simulink model "CraneModel"  (R2021b)
settings: Solver=VariableStepAuto  StartTime=0.0  StopTime=20  MaxStep=0.0001  RelTol=1e-3
values from neighbouring files (symbols this model uses):
  B_x = 12    [variables.m]
  cFrictionX = 18    [variables.m]
  InitWireLength = 1    [variables.m]
  InitXPos = 0    [variables.m]
  J_x = 0.13    [variables.m]
  k_ex = 0.609    [variables.m]
  m_l = 3.89    [variables.m]
  m_t = 0.729    [variables.m]
  r_x = 0.075    [variables.m]
  sFrictionX = 20    [variables.m]
settings Model: Creator=laula  LastModifiedBy=bosto

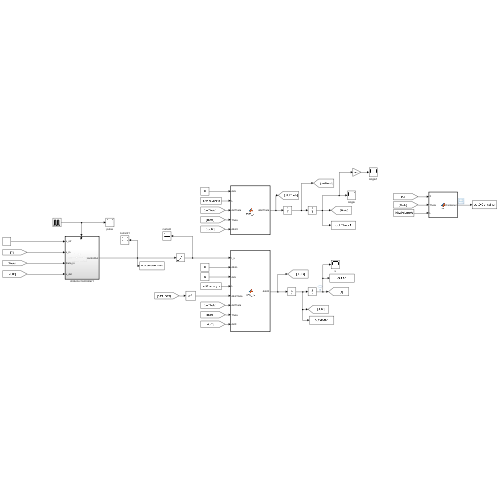
[thumbnail: Simulink's stored preview of the top-level diagram]
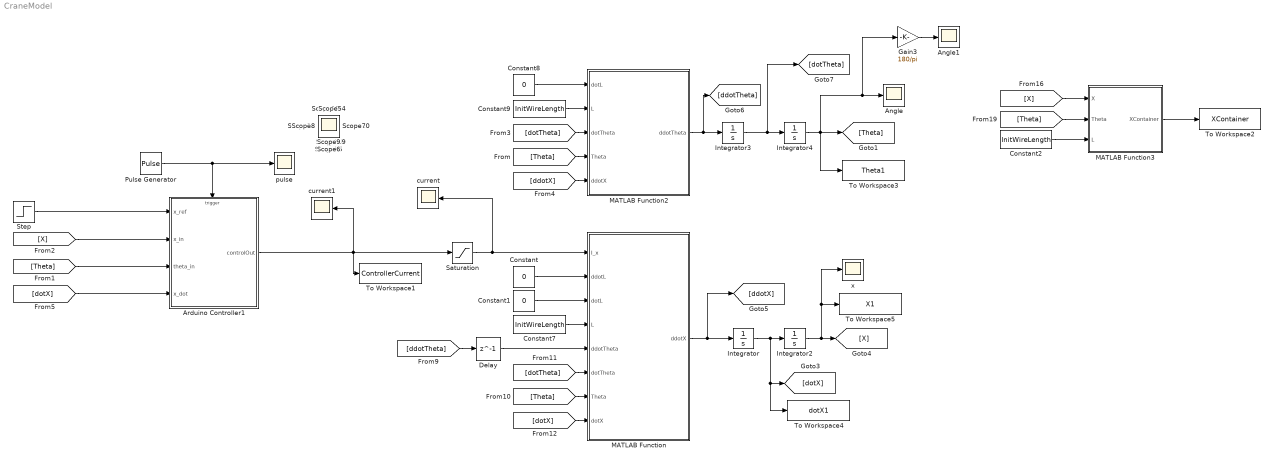
== system CraneModel ==
  Angle : Scope
  Angle1 : Scope
  Arduino Controller1 : Subsystem
  Constant : Constant  Value=0
  Constant1 : Constant  Value=0
  Constant2 : Constant  Value=InitWireLength
  Constant7 : Constant  Value=InitWireLength
  Constant8 : Constant  Value=0
  Constant9 : Constant  Value=InitWireLength
  Delay : Delay  DelayLength=1  InitialCondition=0
  Gain3 : Gain  Gain=180/pi
  Integrator : Integrator
  Integrator2 : Integrator  InitialCondition=InitXPos
  Integrator3 : Integrator
  Integrator4 : Integrator
  MATLAB Function : MATLAB Function  TreatAsAtomicUnit=on
  MATLAB Function2 : MATLAB Function  TreatAsAtomicUnit=on
  MATLAB Function3 : MATLAB Function  TreatAsAtomicUnit=on
  Pulse Generator : DiscretePulseGenerator  PulseType=Time based  Period=.01  PulseWidth=5
  Saturation : Saturate  UpperLimit=10  LowerLimit=-10
  Step : Step  After=3  SampleTime=0
  To Workspace1 : ToWorkspace  VariableName=ControllerCurrent  SampleTime=-1
  To Workspace2 : ToWorkspace  VariableName=XContainer  SampleTime=-1
  To Workspace3 : ToWorkspace  VariableName=Theta1  SampleTime=-1
  To Workspace4 : ToWorkspace  VariableName=dotX1  SampleTime=-1
  To Workspace5 : ToWorkspace  VariableName=X1  SampleTime=-1
  current : Scope
  current1 : Scope
  pulse : Scope
  x : Scope
  Scope{,1..20} (21 alike) : Scope
  wires:
  Constant8/1 -> MATLAB Function2/1(dotL)
  Constant9/1 -> MATLAB Function2/2(L)
  [dotTheta] -> MATLAB Function2/3(dotTheta)
  [Theta] -> MATLAB Function2/4(Theta)
  [ddotX] -> MATLAB Function2/5(ddotX)
  Constant/1 -> MATLAB Function/2(ddotL)
  Constant1/1 -> MATLAB Function/3(dotL)
  Constant7/1 -> MATLAB Function/4(L)
  [dotTheta] -> MATLAB Function/6(dotTheta)
  [Theta] -> MATLAB Function/7(Theta)
  [dotX] -> MATLAB Function/8(dotX)
  Constant2/1 -> MATLAB Function3/3(L)
  [X] -> MATLAB Function3/1(X)
  [Theta] -> MATLAB Function3/2(Theta)
  MATLAB Function3/1(XContainer) -> To Workspace2/1
  MATLAB Function/1(ddotX) -> [ddotX], Integrator/1
  Integrator/1 -> To Workspace4/1, [dotX], Integrator2/1
  Integrator2/1 -> x/1, To Workspace5/1, [X]
  MATLAB Function2/1(ddotTheta) -> [ddotTheta], Integrator3/1
  Integrator3/1 -> [dotTheta], Integrator4/1
  Integrator4/1 -> Gain3/1, Angle/1, To Workspace3/1, [Theta]
  [ddotTheta] -> Delay/1
  Delay/1 -> MATLAB Function/5(ddotTheta)
  Saturation/1 -> current/1, MATLAB Function/1(I_x)
  Step/1 -> Arduino Controller1/1(x_ref)
  Pulse Generator/1 -> pulse/1, Arduino Controller1/Trigger
  Arduino Controller1/1(controlOut) -> To Workspace1/1, current1/1, Saturation/1
  [dotX] -> Arduino Controller1/4(x_dot)
  [Theta] -> Arduino Controller1/3(theta_in)
  [X] -> Arduino Controller1/2(x_in)
  Gain3/1 -> Angle1/1

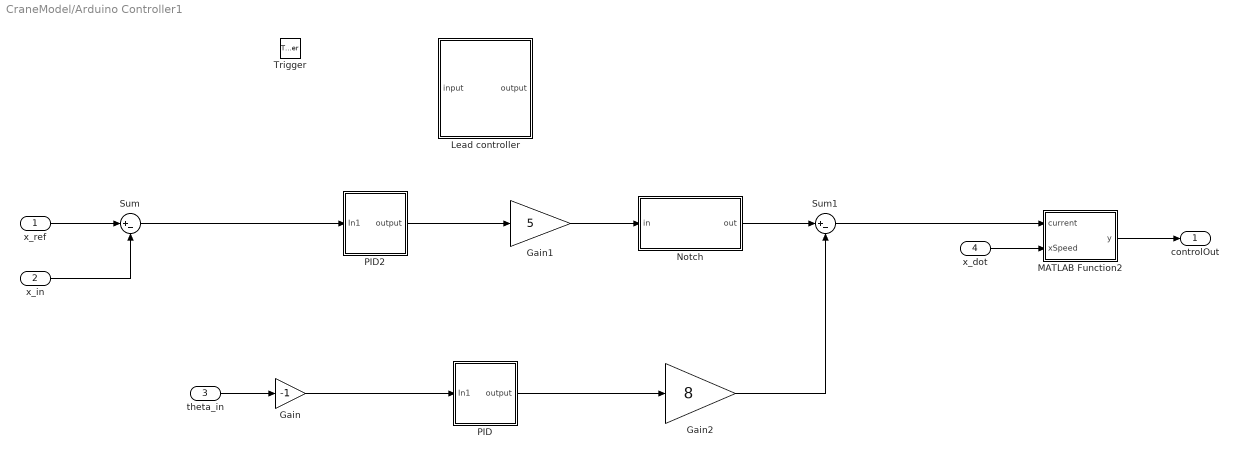
== system CraneModel/Arduino Controller1 ==
  x_ref : Inport
  x_in : Inport  Port=2
  theta_in : Inport  Port=3
  x_dot : Inport  Port=4
  Trigger : TriggerPort  VariantControl=(inherit)  PortDimensions=1
  Gain : Gain  Gain=-1
  Gain1 : Gain  Gain=5
  Gain2 : Gain  Gain=8
  Lead controller : Subsystem
  MATLAB Function2 : MATLAB Function  TreatAsAtomicUnit=on
  Notch : Subsystem
  PID : Subsystem
  PID2 : Subsystem
  Sum : Sum  Inputs=|+-
  Sum1 : Sum  Inputs=|+-
  controlOut : Outport
  wires:
  x_in/1 -> Sum/2
  theta_in/1 -> Gain/1
  x_ref/1 -> Sum/1
  MATLAB Function2/1(y) -> controlOut/1
  Sum1/1 -> MATLAB Function2/1(current)
  x_dot/1 -> MATLAB Function2/2(xSpeed)
  Gain2/1 -> Sum1/2
  Sum/1 -> PID2/1(In1)
  Gain/1 -> PID/1(In1)
  PID/1(output) -> Gain2/1
  PID2/1(output) -> Gain1/1
  Gain1/1 -> Notch/1(in)
  Notch/1(out) -> Sum1/1

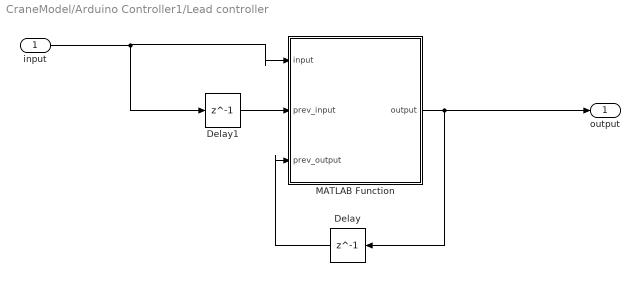
== system CraneModel/Arduino Controller1/Lead controller ==
  input : Inport
  Delay : Delay  DelayLength=1  InitialCondition=0
  Delay1 : Delay  DelayLength=1  InitialCondition=0
  MATLAB Function : MATLAB Function  TreatAsAtomicUnit=on
  output : Outport
  wires:
  Delay1/1 -> MATLAB Function/2(prev_input)
  Delay/1 -> MATLAB Function/3(prev_output)
  input/1 -> MATLAB Function/1(input), Delay1/1
  MATLAB Function/1(output) -> Delay/1, output/1

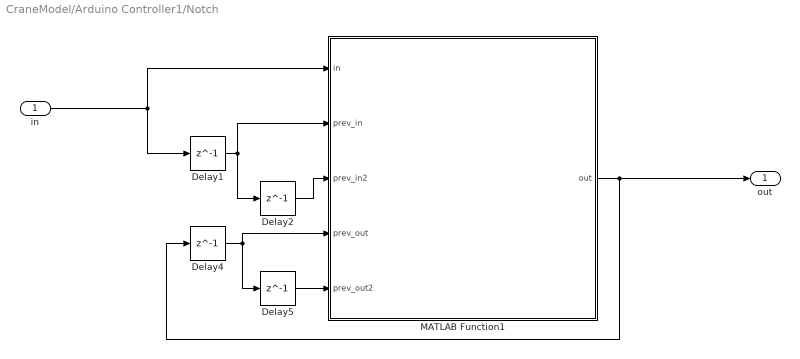
== system CraneModel/Arduino Controller1/Notch ==
  in : Inport
  Delay{1..2,4..5} (4 alike) : Delay  DelayLength=1  InitialCondition=0
  MATLAB Function1 : MATLAB Function  TreatAsAtomicUnit=on
  out : Outport
  wires:
  Delay1/1 -> Delay2/1, MATLAB Function1/2(prev_in)
  MATLAB Function1/1(out) -> out/1, Delay4/1
  Delay2/1 -> MATLAB Function1/3(prev_in2)
  in/1 -> Delay1/1, MATLAB Function1/1(in)
  Delay5/1 -> MATLAB Function1/5(prev_out2)
  Delay4/1 -> Delay5/1, MATLAB Function1/4(prev_out)

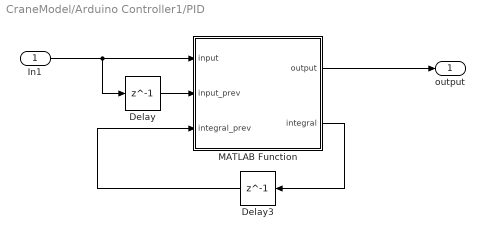
== system CraneModel/Arduino Controller1/PID ==
  In1 : Inport
  Delay : Delay  DelayLength=1  InitialCondition=0
  Delay3 : Delay  DelayLength=1  InitialCondition=0
  MATLAB Function : MATLAB Function  TreatAsAtomicUnit=on
  output : Outport
  wires:
  MATLAB Function/2(integral) -> Delay3/1
  In1/1 -> Delay/1, MATLAB Function/1(input)
  Delay3/1 -> MATLAB Function/3(integral_prev)
  Delay/1 -> MATLAB Function/2(input_prev)
  MATLAB Function/1(output) -> output/1

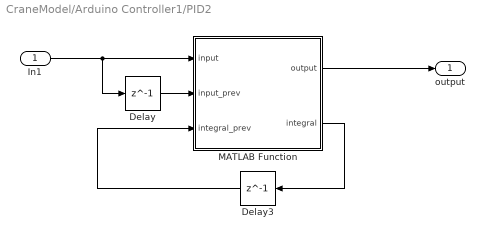
== system CraneModel/Arduino Controller1/PID2 ==
  In1 : Inport
  Delay : Delay  DelayLength=1  InitialCondition=0
  Delay3 : Delay  DelayLength=1  InitialCondition=0
  MATLAB Function : MATLAB Function  TreatAsAtomicUnit=on
  output : Outport
  wires:
  MATLAB Function/2(integral) -> Delay3/1
  In1/1 -> Delay/1, MATLAB Function/1(input)
  Delay3/1 -> MATLAB Function/3(integral_prev)
  Delay/1 -> MATLAB Function/2(input_prev)
  MATLAB Function/1(output) -> output/1

== matlab function CraneModel/Arduino Controller1/MATLAB Function2 ==
  data: current input; y output; xSpeed input
function y = fcn(current, xSpeed)
    if (abs(current) < 0.3)
        y = 0;
    elseif (xSpeed < 0)
        y = current - 2.8;
    
    elseif (xSpeed > 0)
        y = current + 2.8;
    else 
        y = current;
    end
end

== matlab function CraneModel/Arduino Controller1/PID2/MATLAB Function ==
  data: input input; output output; input_prev input; integral_prev input; integral output
function [output, integral]= parallelPID(input, input_prev, integral_prev)
P = 1;
I = 0;
D = 1;
deltaTime = .01;

proportional = input*P;
derivative = D*(input-input_prev)/deltaTime;
integral = integral_prev + I*input*deltaTime; 

output = proportional+derivative+integral;

end

== matlab function CraneModel/Arduino Controller1/Lead controller/MATLAB Function ==
  data: input input; output output; prev_input input; prev_output input
function output = fcn(input, prev_input, prev_output)
    a = 1;
    b = 4;
    k = b/a;   
    dtime = .01;

    output = (k*(input*(1+a*dtime)-prev_input)+prev_output)/(1+b*(dtime));

== matlab function CraneModel/MATLAB Function ==
  data: I_x input; ddotX output; ddotL input; dotL input; L input; ddotTheta input; dotTheta input; Theta input; dotX input; J_x parameter; r_x parameter double; k_ex parameter; m_t parameter; m_l parameter; B_x parameter; sFrictionX parameter; cFrictionX parameter
function ddotX = fcn5_10(I_x, ddotL, dotL, L, ddotTheta, dotTheta, Theta, dotX, J_x, r_x, k_ex, m_t, m_l, B_x,sFrictionX, cFrictionX)

if(norm(dotX)<0.05)
    friction = sFrictionX*sign(dotX);
else
    friction = B_x*dotX+cFrictionX*sign(dotX);
end



temp = I_x*k_ex/r_x;

temp = temp  - m_l*ddotL*sin(Theta);

temp= temp -2*m_l*dotL*dotTheta*cos(Theta);

temp = temp - m_l*L*ddotTheta*cos(Theta);

temp = temp + m_l*L*(dotTheta^2)*sin(Theta);

temp = temp - friction;

temp = temp/(m_t+m_l+J_x/(r_x^2));

ddotX = temp;

== matlab function CraneModel/MATLAB Function2 ==
  data: ddotTheta output; dotL input; L input; dotTheta input; Theta input; ddotX input; g parameter
function ddotTheta = fcn5_7(dotL, L, dotTheta, Theta,ddotX,g)

temp = -2*dotL*dotTheta;

temp = temp - ddotX*cos(Theta);

temp = temp - g*sin(Theta);

temp = temp/L;

ddotTheta = temp;

== matlab function CraneModel/MATLAB Function3 ==
  data: X input; XContainer output; Theta input; L input
function XContainer = fcn(X,Theta,L)

XContainer = X + sin(Theta)*L;

== matlab function CraneModel/Arduino Controller1/Notch/MATLAB Function1 ==
  data: in input; out output; prev_in input; prev_in2 input; prev_out input; prev_out2 input
function out = fcn(in, prev_in, prev_in2, prev_out, prev_out2)

freq = 2/.01*tan(3.14*0.1/2);

b0 = freq^2*.01^2+4;
b1 = 2*freq^2*.01^2+8;
b2 = b0;
a0 = 2*freq*.01 + b0;
a1 = b1;
a2 = -2*freq*.01 + b0;

output = in*b0+ prev_in*b1+ prev_in2*b2- prev_out*a1- prev_out2*a2 ;

    output = output/a0;

    out = output;

== matlab function CraneModel/Arduino Controller1/PID/MATLAB Function ==
  data: input input; output output; input_prev input; integral_prev input; integral output
function [output, integral]= parallelPID(input, input_prev, integral_prev)
P = .25;
I = 0;
D = 1;
deltaTime = .01;

proportional = input*P;
derivative = D*(input-input_prev)/deltaTime;
integral = integral_prev + I*input*deltaTime; 

output = proportional+derivative+integral;

end
